simulink model "car"  (R2016a)
settings: Solver=VariableStepAuto  StartTime=0.0  StopTime=10.0  RelTol=1e-3
libraries: simulink x1
settings Model: Creator=richa  LastModifiedBy=richa

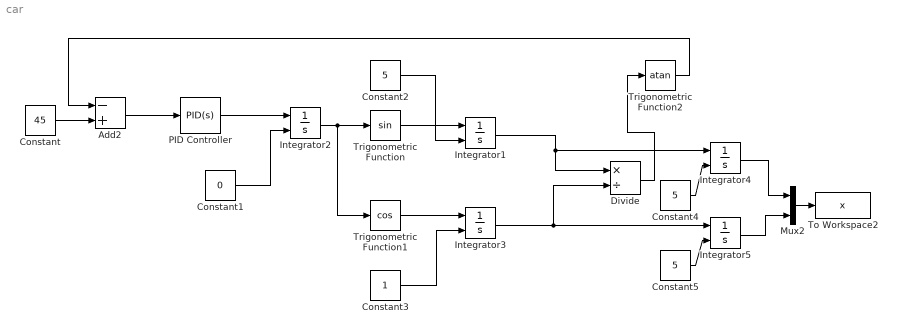
== system car ==
  Add2 : Sum  Inputs=-+
  Constant : Constant  Value=45
  Constant1 : Constant  Value=0
  Constant2 : Constant  Value=5
  Constant3 : Constant
  Constant4 : Constant  Value=5
  Constant5 : Constant  Value=5
  Divide : Product  Inputs=*/
  Integrator{1..5} (5 alike) : Integrator  InitialConditionSource=external
  Mux2 : Mux  Inputs=2
  PID Controller : simulink/Continuous/PID Controller  Controller=PID  TimeDomain=Continuous-time  SampleTime=-1  IntegratorMethod=Forward Euler  FilterMethod=Forward Euler  Form=Parallel  UseFilter=on  ControllerParametersSource=internal  P=1  I=1  D=0  N=100  InitialConditionSource=internal  InitialConditionForIntegrator=0  InitialConditionForFilter=0  ExternalReset=none  LimitOutput=off  UpperSaturationLimit=inf  LowerSaturationLimit=-inf  LinearizeAsGain=on  AntiWindupMode=none  Kb=1  TrackingMode=off  Kt=1  PParamMin=[]  PParamMax=[]  IParamMin=[]  IParamMax=[]  DParamMin=[]  DParamMax=[]  NParamMin=[]  NParamMax=[]  KbParamMin=[]  KbParamMax=[]  KtParamMin=[]  KtParamMax=[]  POutMin=[]  POutMax=[]  IOutMin=[]  IOutMax=[]  DOutMin=[]  DOutMax=[]  NOutMin=[]  NOutMax=[]  KbOutMin=[]  KbOutMax=[]  KtOutMin=[]  KtOutMax=[]  IntegratorOutMin=[]  IntegratorOutMax=[]  FilterOutMin=[]  FilterOutMax=[]  SumOutMin=[]  SumOutMax=[]  SumI1OutMin=[]  SumI1OutMax=[]  SumI2OutMin=[]  SumI2OutMax=[]  SumI3OutMin=[]  SumI3OutMax=[]  SumDOutMin=[]  SumDOutMax=[]  SaturationOutMin=[]  SaturationOutMax=[]  IntegratorContinuousStateAttributes=''  IntegratorStateMustResolveToSignalObject=off  IntegratorRTWStateStorageClass=Auto  FilterContinuousStateAttributes=''  FilterStateMustResolveToSignalObject=off  FilterRTWStateStorageClass=Auto  DifferentiatorICPrevScaledInput=0  DifferentiatorOutMin=[]  DifferentiatorOutMax=[]
  To Workspace2 : ToWorkspace  VariableName=x  SampleTime=-1
  Trigonometric Function : Trigonometry
  Trigonometric Function1 : Trigonometry  Operator=cos
  Trigonometric Function2 : Trigonometry  Operator=atan
  wires:
  Add2/1 -> PID Controller/1
  PID Controller/1 -> Integrator2/1
  Integrator2/1 -> Trigonometric Function1/1, Trigonometric Function/1
  Divide/1 -> Trigonometric Function2/1
  Trigonometric Function2/1 -> Add2/1
  Mux2/1 -> To Workspace2/1
  Constant/1 -> Add2/2
  Constant1/1 -> Integrator2/2
  Trigonometric Function/1 -> Integrator1/1
  Integrator1/1 -> Integrator4/1, Divide/1
  Trigonometric Function1/1 -> Integrator3/1
  Integrator3/1 -> Integrator5/1, Divide/2
  Constant2/1 -> Integrator1/2
  Constant3/1 -> Integrator3/2
  Constant4/1 -> Integrator4/2
  Constant5/1 -> Integrator5/2
  Integrator4/1 -> Mux2/1
  Integrator5/1 -> Mux2/2
